simulink subsystem "SMC_Subsystem"  (R2023a)
settings: Solver=VariableStepAuto  StartTime=0.0  StopTime=10.0  RelTol=1e-3

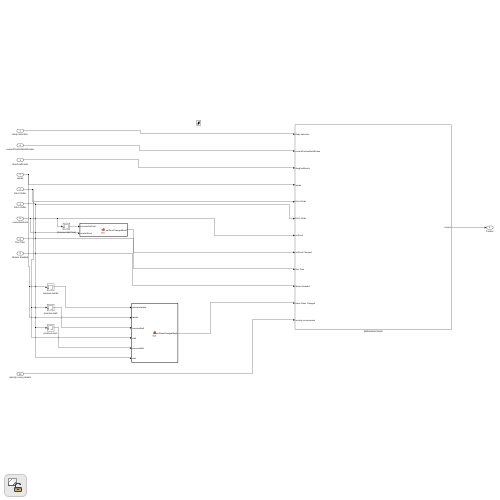
[thumbnail: Simulink's stored preview of the top-level diagram]
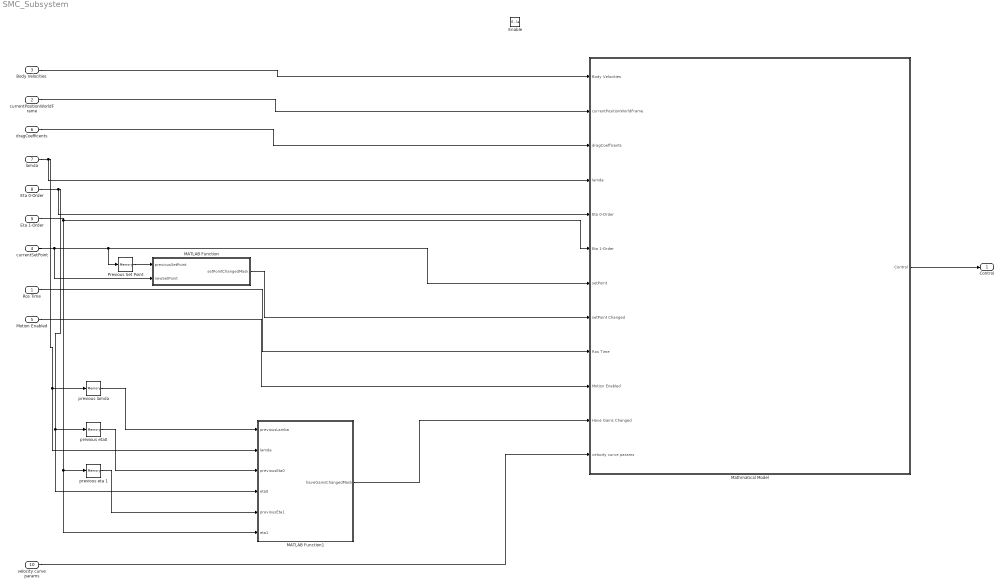
== system SMC_Subsystem ==
  Ros Time : Inport
  currentPositionWorldFrame : Inport  Port=2
  Body Velocities : Inport  Port=3
  currentSetPoint : Inport  Port=4
  Motion Enabled : Inport  Port=5
  dragCoefficents : Inport  Port=6
  lamda : Inport  Port=7
  Eta 0-Order : Inport  Port=8
  Eta 1-Order : Inport  Port=9
  velocity curve params : Inport  Port=10
  Enable : EnablePort
  MATLAB Function : MATLAB Function  TreatAsAtomicUnit=on
  MATLAB Function1 : MATLAB Function  TreatAsAtomicUnit=on
  Mathmatical Model : Subsystem
  Previous Set Point : Memory  InitialCondition=[0,0,0,0,0,0,0]  InheritSampleTime=on
  previous eta 1 : Memory  InheritSampleTime=on
  previous eta0 : Memory  InheritSampleTime=on
  previous lamda : Memory  InheritSampleTime=on
  Control : Outport
  wires:
  dragCoefficents/1 -> Mathmatical Model/3(dragCoefficents)
  Mathmatical Model/1(Control) -> Control/1
  currentSetPoint/1 -> Mathmatical Model/7(setPoint), Previous Set Point/1, MATLAB Function/2(newSetPoint)
  currentPositionWorldFrame/1 -> Mathmatical Model/2(currentPositionWorldFrame)
  Body Velocities/1 -> Mathmatical Model/1(Body Velocities)
  MATLAB Function/1(setPointChangedMask) -> Mathmatical Model/8(setPoint Changed)
  Previous Set Point/1 -> MATLAB Function/1(previousSetPoint)
  Ros Time/1 -> Mathmatical Model/9(Ros Time)
  Motion Enabled/1 -> Mathmatical Model/10(Motion Enabled)
  previous lamda/1 -> MATLAB Function1/1(previousLamba)
  previous eta0/1 -> MATLAB Function1/3(previousEta0)
  previous eta 1/1 -> MATLAB Function1/5(previousEta1)
  lamda/1 -> previous lamda/1, MATLAB Function1/2(lamda), Mathmatical Model/4(lamda)
  Eta 0-Order/1 -> MATLAB Function1/4(eta0), previous eta0/1, Mathmatical Model/5(Eta 0-Order)
  Eta 1-Order/1 -> Mathmatical Model/6(Eta 1-Order), MATLAB Function1/6(eta1), previous eta 1/1
  MATLAB Function1/1(haveGainsChangedMask) -> Mathmatical Model/11(Have Gains Changed)
  velocity curve params/1 -> Mathmatical Model/12(velocity curve params)

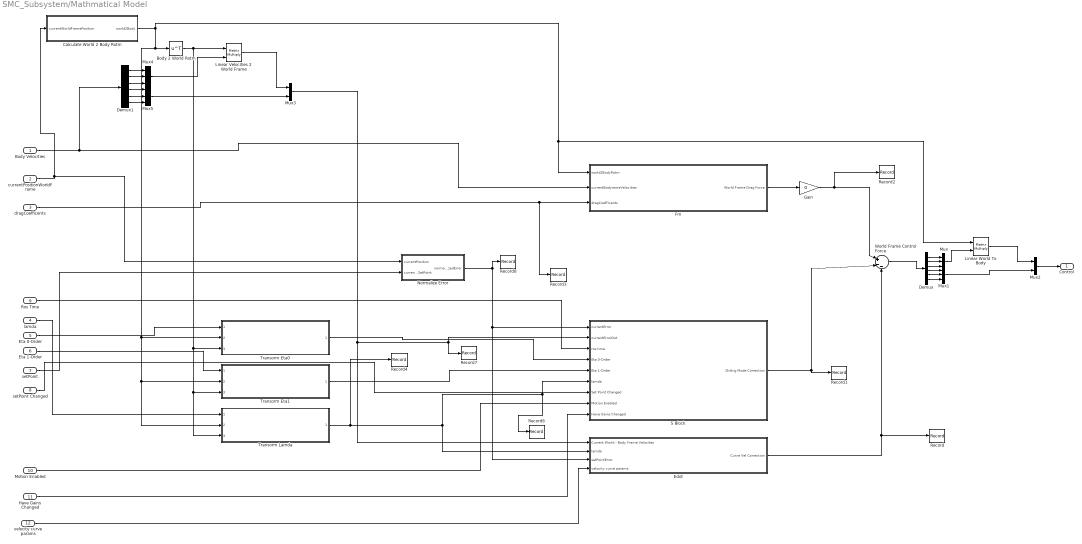
== system SMC_Subsystem/Mathmatical Model ==
  Body Velocities : Inport
  currentPositionWorldFrame : Inport  Port=2
  dragCoefficents : Inport  Port=3
  lamda : Inport  Port=4
  Eta 0-Order : Inport  Port=5
  Eta 1-Order : Inport  Port=6
  setPoint : Inport  Port=7
  setPoint Changed : Inport  Port=8
  Ros Time : Inport  Port=9
  Motion Enabled : Inport  Port=10
  Have Gains Changed : Inport  Port=11
  velocity curve params : Inport  Port=12
  Body 2 World Rotm : Math  Operator=transpose
  Calculate World 2 Body Rotm : MATLAB Function  TreatAsAtomicUnit=on
  Demux : Demux  Outputs=6
  Demux1 : Demux  Outputs=6
  Edot : Subsystem
  Fm : Subsystem
  Gain : Gain  Gain=0
  Linear Velocities 2 World Frame : Product  Multiplication=Matrix(*)
  Linear World To Body : Product  Multiplication=Matrix(*)
  Mux{,1,4..5} (4 alike) : Mux  Inputs=3
  Mux2 : Mux  Inputs=2
  Mux3 : Mux  Inputs=2
  Normalize Error : MATLAB Function  TreatAsAtomicUnit=on
  Record : Record  FileSettingsInternal="{\"entries\":[{\"content\":{\"excelSettings\":{\"content\":{},\"type\":\"Streamout.ExcelSettings\"}},\"type\":\"Streamout.FileSettingStorage\",\"uuid\":\"\"}],\"packageUris\":[\"http:\\/\\/schema.mathworks.com\\/mf0\\/streamout_blocks\\/R2020a\"],\"version\":\"1.0\"}"  Layout=[1 1]  SignalsInternal="{\"entries\":[{\"content\":{\"signals\":[{\"content\":{\"blockPath\":[],\"dimensions\":[6,1],\"domain\":\"\",\"hasChildren\":true,\"lineColor\":\"#b746ff\",\"port\":1,\"signalID\":2555,\"signalName\":\"Edot\"},\"type\":\"RecordBlkView.Signal\",\"uuid\":\"\"},{\"content\":{\"blockPath\":[],\"channel\":[1,1],\"dimensions\":[6,1],\"domain\":\"\",\"lineColor\":\"#4dbeee\",\"parentID\":2555,\"port\":1,\"signalID\":2556,\"signalName\":\"Edot\"},\"type\":\"RecordBlkView ...(+1172 chars)"  VisualizationBindings="{\"sparklinesplugin\":{\"info\":[{\"bindingParametersList\":[],\"subplotID\":1}]}}"
  Record1 : Record  FileSettingsInternal="{\"entries\":[{\"content\":{\"excelSettings\":{\"content\":{},\"type\":\"Streamout.ExcelSettings\"}},\"type\":\"Streamout.FileSettingStorage\",\"uuid\":\"\"}],\"packageUris\":[\"http:\\/\\/schema.mathworks.com\\/mf0\\/streamout_blocks\\/R2020a\"],\"version\":\"1.0\"}"  Layout=[1 1]  SignalsInternal="{\"entries\":[{\"content\":{\"signals\":[{\"content\":{\"blockPath\":[],\"dimensions\":[6,1],\"domain\":\"\",\"hasChildren\":true,\"lineColor\":\"#ff13a6\",\"port\":1,\"signalID\":2572,\"signalName\":\"S Block\"},\"type\":\"RecordBlkView.Signal\",\"uuid\":\"\"},{\"content\":{\"blockPath\":[],\"channel\":[1,1],\"dimensions\":[6,1],\"domain\":\"\",\"lineColor\":\"#0072bd\",\"parentID\":2572,\"port\":1,\"signalID\":2573,\"signalName\":\"S Block\"},\"type\":\"RecordB ...(+1193 chars)"  VisualizationBindings="{\"sparklinesplugin\":{\"info\":[{\"bindingParametersList\":[],\"subplotID\":1}]}}"
  Record2 : Record  FileSettingsInternal="{\"entries\":[{\"content\":{\"excelSettings\":{\"content\":{},\"type\":\"Streamout.ExcelSettings\"}},\"type\":\"Streamout.FileSettingStorage\",\"uuid\":\"\"}],\"packageUris\":[\"http:\\/\\/schema.mathworks.com\\/mf0\\/streamout_blocks\\/R2020a\"],\"version\":\"1.0\"}"  Layout=[1 1]  SignalsInternal="{\"entries\":[{\"content\":{\"signals\":[{\"content\":{\"blockPath\":[],\"dimensions\":[6],\"domain\":\"\",\"hasChildren\":true,\"lineColor\":\"#22b573\",\"port\":1,\"signalID\":2589,\"signalName\":\"Gain\"},\"type\":\"RecordBlkView.Signal\",\"uuid\":\"\"},{\"content\":{\"blockPath\":[],\"channel\":[1],\"dimensions\":[6],\"domain\":\"\",\"lineColor\":\"#edb120\",\"parentID\":2589,\"plots\":[1],\"port\":1,\"signalID\":2590,\"signalName\":\"Gain\"},\"type\":\"RecordB ...(+1206 chars)"  VisualizationBindings="{\"sparklinesplugin\":{\"info\":[{\"bindingParametersList\":[],\"subplotID\":1}]}}"
  Record3 : Record  FileSettingsInternal="{\"entries\":[{\"content\":{\"excelSettings\":{\"content\":{},\"type\":\"Streamout.ExcelSettings\"}},\"type\":\"Streamout.FileSettingStorage\",\"uuid\":\"\"}],\"packageUris\":[\"http:\\/\\/schema.mathworks.com\\/mf0\\/streamout_blocks\\/R2020a\"],\"version\":\"1.0\"}"  Layout=[1 1]  SignalsInternal="{\"entries\":[{\"content\":{\"signals\":[{\"content\":{\"blockPath\":[],\"dimensions\":[1,24],\"domain\":\"\",\"hasChildren\":true,\"lineColor\":\"#d95319\",\"port\":1,\"signalID\":2606,\"signalName\":\"dragCoefficents\"},\"type\":\"RecordBlkView.Signal\",\"uuid\":\"\"},{\"content\":{\"blockPath\":[],\"channel\":[1,1],\"dimensions\":[1,24],\"domain\":\"\",\"lineColor\":\"#77ac30\",\"parentID\":2606,\"plots\":[1],\"port\":1,\"signalID\":2607,\"signalName\":\"dra ...(+5141 chars)"  VisualizationBindings="{\"sparklinesplugin\":{\"info\":[{\"bindingParametersList\":[],\"subplotID\":1}]}}"
  Record4 : Record  FileSettingsInternal="{\"entries\":[{\"content\":{\"excelSettings\":{\"content\":{},\"type\":\"Streamout.ExcelSettings\"}},\"type\":\"Streamout.FileSettingStorage\",\"uuid\":\"\"}],\"packageUris\":[\"http:\\/\\/schema.mathworks.com\\/mf0\\/streamout_blocks\\/R2020a\"],\"version\":\"1.0\"}"  Layout=[1 1]  SignalsInternal="{\"entries\":[{\"content\":{\"signals\":[{\"content\":{\"blockPath\":[],\"dimensions\":[6],\"domain\":\"\",\"hasChildren\":true,\"lineColor\":\"#7e2f8e\",\"port\":1,\"signalID\":2659,\"signalName\":\"Transorm Lamda\"},\"type\":\"RecordBlkView.Signal\",\"uuid\":\"\"},{\"content\":{\"blockPath\":[],\"channel\":[1],\"dimensions\":[6],\"domain\":\"\",\"lineColor\":\"#64d413\",\"parentID\":2659,\"plots\":[1],\"port\":1,\"signalID\":2660,\"signalName\":\"Transorm Lam ...(+1276 chars)"  VisualizationBindings="{\"sparklinesplugin\":{\"info\":[{\"bindingParametersList\":[],\"subplotID\":1}]}}"
  Record6 : Record  FileSettingsInternal="{\"entries\":[{\"content\":{\"excelSettings\":{\"content\":{},\"type\":\"Streamout.ExcelSettings\"}},\"type\":\"Streamout.FileSettingStorage\",\"uuid\":\"\"}],\"packageUris\":[\"http:\\/\\/schema.mathworks.com\\/mf0\\/streamout_blocks\\/R2020a\"],\"version\":\"1.0\"}"  Layout=[1 1]  SignalsInternal="{\"entries\":[{\"content\":{\"signals\":[{\"content\":{\"blockPath\":[],\"dimensions\":[6],\"domain\":\"\",\"hasChildren\":true,\"lineColor\":\"#4dbeee\",\"port\":1,\"signalID\":2676,\"signalName\":\"Transorm Lamda\"},\"type\":\"RecordBlkView.Signal\",\"uuid\":\"\"},{\"content\":{\"blockPath\":[],\"channel\":[1],\"dimensions\":[6],\"domain\":\"\",\"lineColor\":\"#64d413\",\"parentID\":2676,\"plots\":[1],\"port\":1,\"signalID\":2677,\"signalName\":\"Transorm Lam ...(+1240 chars)"  VisualizationBindings="{\"sparklinesplugin\":{\"info\":[{\"bindingParametersList\":[],\"subplotID\":1}]}}"
  Record7 : Record  FileSettingsInternal="{\"entries\":[{\"content\":{\"excelSettings\":{\"content\":{},\"type\":\"Streamout.ExcelSettings\"}},\"type\":\"Streamout.FileSettingStorage\",\"uuid\":\"\"}],\"packageUris\":[\"http:\\/\\/schema.mathworks.com\\/mf0\\/streamout_blocks\\/R2020a\"],\"version\":\"1.0\"}"  Layout=[1 1]  SignalsInternal="{\"entries\":[{\"content\":{\"signals\":[{\"content\":{\"blockPath\":[],\"dimensions\":[6],\"domain\":\"\",\"hasChildren\":true,\"lineColor\":\"#139fff\",\"port\":1,\"signalID\":2693,\"signalName\":\"Mux3\"},\"type\":\"RecordBlkView.Signal\",\"uuid\":\"\"},{\"content\":{\"blockPath\":[],\"channel\":[1],\"dimensions\":[6],\"domain\":\"\",\"lineColor\":\"#edb120\",\"parentID\":2693,\"plots\":[1],\"port\":1,\"signalID\":2694,\"signalName\":\"Mux3\"},\"type\":\"RecordB ...(+1170 chars)"  VisualizationBindings="{\"sparklinesplugin\":{\"info\":[{\"bindingParametersList\":[],\"subplotID\":1}]}}"
  Record8 : Record  FileSettingsInternal="{\"entries\":[{\"content\":{\"excelSettings\":{\"content\":{},\"type\":\"Streamout.ExcelSettings\"}},\"type\":\"Streamout.FileSettingStorage\",\"uuid\":\"\"}],\"packageUris\":[\"http:\\/\\/schema.mathworks.com\\/mf0\\/streamout_blocks\\/R2020a\"],\"version\":\"1.0\"}"  Layout=[1 1]  SignalsInternal="{\"entries\":[{\"content\":{\"signals\":[{\"content\":{\"blockPath\":[],\"dimensions\":[1,6],\"domain\":\"\",\"hasChildren\":true,\"lineColor\":\"#b746ff\",\"port\":1,\"signalID\":2710,\"signalName\":\"Normalize Error\"},\"type\":\"RecordBlkView.Signal\",\"uuid\":\"\"},{\"content\":{\"blockPath\":[],\"channel\":[1,1],\"dimensions\":[1,6],\"domain\":\"\",\"lineColor\":\"#a2142f\",\"parentID\":2710,\"plots\":[1],\"port\":1,\"signalID\":2711,\"signalName\":\"Norma ...(+1273 chars)"  VisualizationBindings="{\"sparklinesplugin\":{\"info\":[{\"bindingParametersList\":[],\"subplotID\":1}]}}"
  S Block : Subsystem
  Transorm Eta0 : Subsystem  ReferencedSubsystem=Tranfsform_Linear_Gains_To_World
  Transorm Eta1 : Subsystem  ReferencedSubsystem=Tranfsform_Linear_Gains_To_World
  Transorm Lamda : Subsystem  ReferencedSubsystem=Tranfsform_Linear_Gains_To_World
  World Frame Control Force : Sum  Inputs=|+--
  Control : Outport
  wires:
  velocity curve params/1 -> Edot/4(velocity curve params)
  Have Gains Changed/1 -> S Block/9(Have Gains Changed)
  Motion Enabled/1 -> S Block/8(Motion Enabled)
  Transorm Eta0/1 -> S Block/4(Eta 0-Order)
  Body 2 World Rotm/1 -> Linear Velocities 2 World Frame/1, Transorm Lamda/3, Transorm Eta1/3, Transorm Eta0/3
  Edot/1(Curve Vel Correction) -> World Frame Control Force/3, Record/1
  Gain/1 -> World Frame Control Force/1, Record2/1
  Eta 1-Order/1 -> Transorm Eta1/1
  setPoint/1 -> Normalize Error/2(currentSetPoint)
  Normalize Error/1(normalizedError) -> S Block/1(currentError), Edot/3(setPointError), Record8/1
  Ros Time/1 -> S Block/3(ros time)
  setPoint Changed/1 -> S Block/7(Set Point Changed)
  Mux3/1 -> Edot/1(Current World - Body Frame Velocites), S Block/2(currentErrorDot), Record7/1
  Eta 0-Order/1 -> Transorm Eta0/1
  lamda/1 -> Transorm Lamda/1
  Transorm Eta1/1 -> S Block/5(Eta 1-Order)
  Transorm Lamda/1 -> Edot/2(lamda), S Block/6(lamda), Record6/1, Record4/1
  Mux5/1 -> Mux3/2
  Fm/1(World Frame Drag Force) -> Gain/1
  Demux1/6 -> Mux5/3
  Demux1/4 -> Mux5/1
  Demux1/5 -> Mux5/2
  Demux1/3 -> Mux4/3
  Demux1/1 -> Mux4/1
  Demux1/2 -> Mux4/2
  Mux4/1 -> Linear Velocities 2 World Frame/2
  Linear Velocities 2 World Frame/1 -> Mux3/1
  dragCoefficents/1 -> Fm/3(dragCoefficents), Record3/1
  Calculate World 2 Body Rotm/1(world2Body) -> Fm/1(world2BodyRotm), Linear World To Body/1, Transorm Lamda/2, Transorm Eta1/2, Transorm Eta0/2, Body 2 World Rotm/1
  Mux2/1 -> Control/1
  Mux1/1 -> Mux2/2
  Linear World To Body/1 -> Mux2/1
  Mux/1 -> Linear World To Body/2
  Demux/4 -> Mux1/1
  Demux/5 -> Mux1/2
  Demux/6 -> Mux1/3
  Demux/3 -> Mux/3
  Demux/2 -> Mux/2
  Demux/1 -> Mux/1
  World Frame Control Force/1 -> Demux/1
  S Block/1("Sliding Mode Correction ") -> Record1/1, World Frame Control Force/2
  currentPositionWorldFrame/1 -> Calculate World 2 Body Rotm/1(currentWorldFramePosition), Normalize Error/1(currentPosition)
  Body Velocities/1 -> Demux1/1, Fm/2(currentBodyrameVelocities)

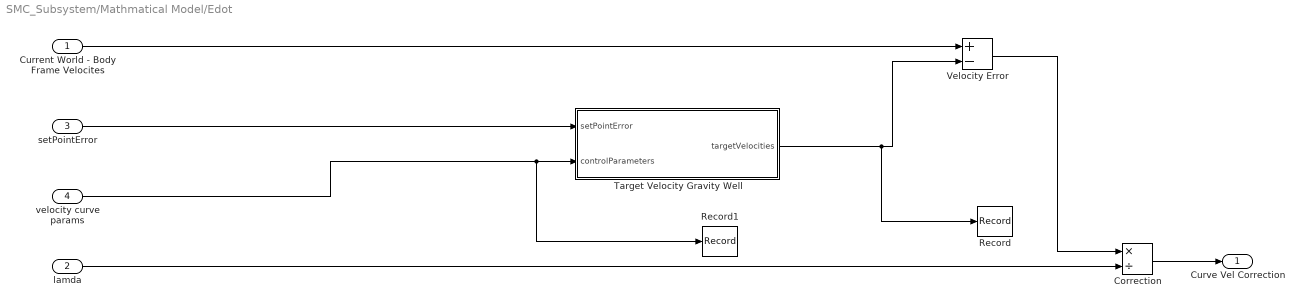
== system SMC_Subsystem/Mathmatical Model/Edot ==
  Current World - Body Frame Velocites : Inport
  lamda : Inport  Port=2
  setPointError : Inport  Port=3
  velocity curve params : Inport  Port=4
  Correction : Product  Inputs=*/
  Record : Record  FileSettingsInternal="{\"entries\":[{\"content\":{\"excelSettings\":{\"content\":{},\"type\":\"Streamout.ExcelSettings\"}},\"type\":\"Streamout.FileSettingStorage\",\"uuid\":\"\"}],\"packageUris\":[\"http:\\/\\/schema.mathworks.com\\/mf0\\/streamout_blocks\\/R2020a\"],\"version\":\"1.0\"}"  Layout=[1 1]  SignalsInternal="{\"entries\":[{\"content\":{\"signals\":[{\"content\":{\"blockPath\":[],\"dimensions\":[6,1],\"domain\":\"\",\"hasChildren\":true,\"lineColor\":\"#ff13a6\",\"port\":1,\"signalID\":2441,\"signalName\":\"Target Velocity Gravity Well\"},\"type\":\"RecordBlkView.Signal\",\"uuid\":\"\"},{\"content\":{\"blockPath\":[],\"channel\":[1,1],\"dimensions\":[6,1],\"domain\":\"\",\"lineColor\":\"#d95319\",\"parentID\":2441,\"plots\":[1],\"port\":1,\"signalID\":2442,\"signa ...(+1340 chars)"  VisualizationBindings="{\"sparklinesplugin\":{\"info\":[{\"bindingParametersList\":[],\"subplotID\":1}]}}"
  Record1 : Record  FileSettingsInternal="{\"entries\":[{\"content\":{\"excelSettings\":{\"content\":{},\"type\":\"Streamout.ExcelSettings\"}},\"type\":\"Streamout.FileSettingStorage\",\"uuid\":\"\"}],\"packageUris\":[\"http:\\/\\/schema.mathworks.com\\/mf0\\/streamout_blocks\\/R2020a\"],\"version\":\"1.0\"}"  Layout=[1 1]  SignalsInternal="{\"entries\":[{\"content\":{\"signals\":[{\"content\":{\"blockPath\":[],\"dimensions\":[1,12],\"domain\":\"\",\"hasChildren\":true,\"lineColor\":\"#22b573\",\"port\":1,\"signalID\":2458,\"signalName\":\"velocity curve params\"},\"type\":\"RecordBlkView.Signal\",\"uuid\":\"\"},{\"content\":{\"blockPath\":[],\"channel\":[1,1],\"dimensions\":[1,12],\"domain\":\"\",\"lineColor\":\"#edb120\",\"parentID\":2458,\"plots\":[1],\"port\":1,\"signalID\":2459,\"signalName ...(+2639 chars)"  VisualizationBindings="{\"sparklinesplugin\":{\"info\":[{\"bindingParametersList\":[],\"subplotID\":1}]}}"
  Target Velocity Gravity Well : MATLAB Function  TreatAsAtomicUnit=on
  Velocity Error : Sum  Inputs=+-
  Curve Vel Correction : Outport
  wires:
  velocity curve params/1 -> Target Velocity Gravity Well/2(controlParameters), Record1/1
  Target Velocity Gravity Well/1(targetVelocities) -> Velocity Error/2, Record/1
  setPointError/1 -> Target Velocity Gravity Well/1(setPointError)
  Velocity Error/1 -> Correction/1
  Current World - Body Frame Velocites/1 -> Velocity Error/1
  lamda/1 -> Correction/2
  Correction/1 -> Curve Vel Correction/1

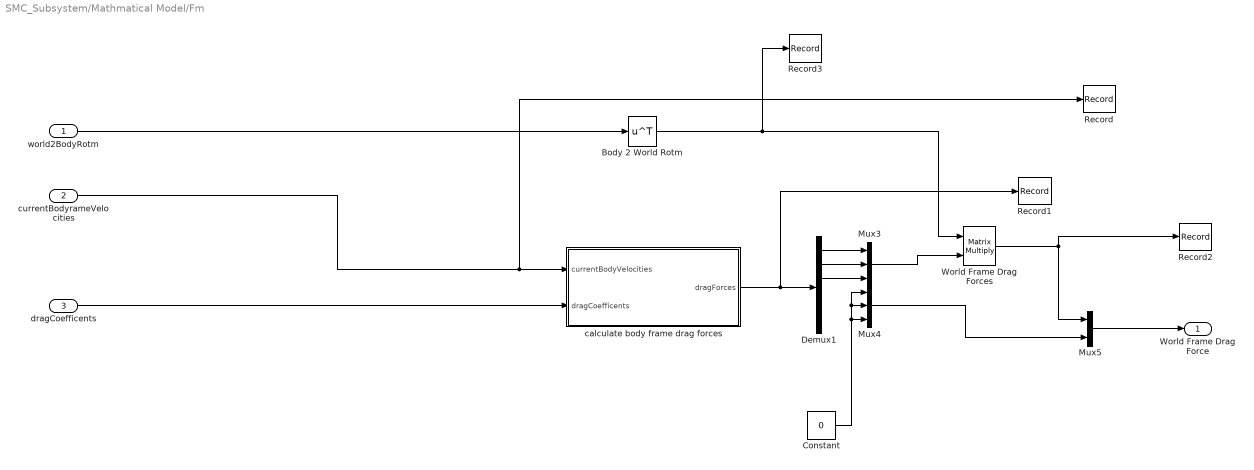
== system SMC_Subsystem/Mathmatical Model/Fm ==
  world2BodyRotm : Inport
  currentBodyrameVelocities : Inport  Port=2
  dragCoefficents : Inport  Port=3
  Body 2 World Rotm : Math  Operator=transpose
  Constant : Constant  Value=0
  Demux1 : Demux  Outputs=6
  Mux3 : Mux  Inputs=3
  Mux4 : Mux  Inputs=3
  Mux5 : Mux  Inputs=2
  Record : Record  FileSettingsInternal="{\"entries\":[{\"content\":{\"excelSettings\":{\"content\":{},\"type\":\"Streamout.ExcelSettings\"}},\"type\":\"Streamout.FileSettingStorage\",\"uuid\":\"\"}],\"packageUris\":[\"http:\\/\\/schema.mathworks.com\\/mf0\\/streamout_blocks\\/R2020a\"],\"version\":\"1.0\"}"  Layout=[1 1]  SignalsInternal="{\"entries\":[{\"content\":{\"signals\":[{\"content\":{\"blockPath\":[],\"dimensions\":[6],\"domain\":\"\",\"hasChildren\":true,\"lineColor\":\"#d95319\",\"port\":1,\"signalID\":2487,\"signalName\":\"currentBodyrameVelocities\"},\"type\":\"RecordBlkView.Signal\",\"uuid\":\"\"},{\"content\":{\"blockPath\":[],\"channel\":[1],\"dimensions\":[6],\"domain\":\"\",\"lineColor\":\"#b746ff\",\"parentID\":2487,\"plots\":[1],\"port\":1,\"signalID\":2488,\"signalName\":\"c ...(+1341 chars)"  VisualizationBindings="{\"sparklinesplugin\":{\"info\":[{\"bindingParametersList\":[],\"subplotID\":1}]}}"
  Record1 : Record  FileSettingsInternal="{\"entries\":[{\"content\":{\"excelSettings\":{\"content\":{},\"type\":\"Streamout.ExcelSettings\"}},\"type\":\"Streamout.FileSettingStorage\",\"uuid\":\"\"}],\"packageUris\":[\"http:\\/\\/schema.mathworks.com\\/mf0\\/streamout_blocks\\/R2020a\"],\"version\":\"1.0\"}"  Layout=[1 1]  SignalsInternal="{\"entries\":[{\"content\":{\"signals\":[{\"content\":{\"blockPath\":[],\"dimensions\":[6,1],\"domain\":\"\",\"hasChildren\":true,\"lineColor\":\"#7e2f8e\",\"port\":1,\"signalID\":2504,\"signalName\":\"calculate body frame drag forces\"},\"type\":\"RecordBlkView.Signal\",\"uuid\":\"\"},{\"content\":{\"blockPath\":[],\"channel\":[1,1],\"dimensions\":[6,1],\"domain\":\"\",\"lineColor\":\"#139fff\",\"parentID\":2504,\"plots\":[1],\"port\":1,\"signalID\":2505,\"s ...(+1428 chars)"  VisualizationBindings="{\"sparklinesplugin\":{\"info\":[{\"bindingParametersList\":[],\"subplotID\":1}]}}"
  Record2 : Record  FileSettingsInternal="{\"entries\":[{\"content\":{\"excelSettings\":{\"content\":{},\"type\":\"Streamout.ExcelSettings\"}},\"type\":\"Streamout.FileSettingStorage\",\"uuid\":\"\"}],\"packageUris\":[\"http:\\/\\/schema.mathworks.com\\/mf0\\/streamout_blocks\\/R2020a\"],\"version\":\"1.0\"}"  SignalsInternal="{\"entries\":[{\"content\":{\"signals\":[{\"content\":{\"blockPath\":[],\"dimensions\":[3],\"domain\":\"\",\"hasChildren\":true,\"lineColor\":\"#4dbeee\",\"port\":1,\"signalID\":2521,\"signalName\":\"World Frame Drag Forces\"},\"type\":\"RecordBlkView.Signal\",\"uuid\":\"\"},{\"content\":{\"blockPath\":[],\"channel\":[1],\"dimensions\":[3],\"domain\":\"\",\"lineColor\":\"#b746ff\",\"parentID\":2521,\"plots\":[1],\"port\":1,\"signalID\":2522,\"signalName\":\"Wor ...(+661 chars)"  VisualizationBindings="{\"sparklinesplugin\":{\"info\":[{\"bindingParametersList\":[],\"subplotID\":1}]}}"
  Record3 : Record  FileSettingsInternal="{\"entries\":[{\"content\":{\"excelSettings\":{\"content\":{},\"type\":\"Streamout.ExcelSettings\"}},\"type\":\"Streamout.FileSettingStorage\",\"uuid\":\"\"}],\"packageUris\":[\"http:\\/\\/schema.mathworks.com\\/mf0\\/streamout_blocks\\/R2020a\"],\"version\":\"1.0\"}"  Layout=[1 1]  SignalsInternal="{\"entries\":[{\"content\":{\"signals\":[{\"content\":{\"blockPath\":[],\"dimensions\":[3,3],\"domain\":\"\",\"hasChildren\":true,\"lineColor\":\"#139fff\",\"port\":1,\"signalID\":2532,\"signalName\":\"Body 2 World Rotm\"},\"type\":\"RecordBlkView.Signal\",\"uuid\":\"\"},{\"content\":{\"blockPath\":[],\"channel\":[1,1],\"dimensions\":[3,3],\"domain\":\"\",\"lineColor\":\"#a2142f\",\"parentID\":2532,\"plots\":[1],\"port\":1,\"signalID\":2533,\"signalName\":\"Bod ...(+1995 chars)"  VisualizationBindings="{\"sparklinesplugin\":{\"info\":[{\"bindingParametersList\":[],\"subplotID\":1}]}}"
  World Frame Drag Forces : Product  Multiplication=Matrix(*)
  calculate body frame drag forces : MATLAB Function  TreatAsAtomicUnit=on
  World Frame Drag Force : Outport
  wires:
  Constant/1 -> Mux4/1, Mux4/2, Mux4/3
  Mux4/1 -> Mux5/2
  calculate body frame drag forces/1(dragForces) -> Demux1/1, Record1/1
  Body 2 World Rotm/1 -> World Frame Drag Forces/1, Record3/1
  world2BodyRotm/1 -> Body 2 World Rotm/1
  dragCoefficents/1 -> calculate body frame drag forces/2(dragCoefficents)
  currentBodyrameVelocities/1 -> calculate body frame drag forces/1(currentBodyVelocities), Record/1
  Demux1/2 -> Mux3/2
  Mux5/1 -> World Frame Drag Force/1
  Demux1/3 -> Mux3/3
  Mux3/1 -> World Frame Drag Forces/2
  Demux1/1 -> Mux3/1
  World Frame Drag Forces/1 -> Record2/1, Mux5/1

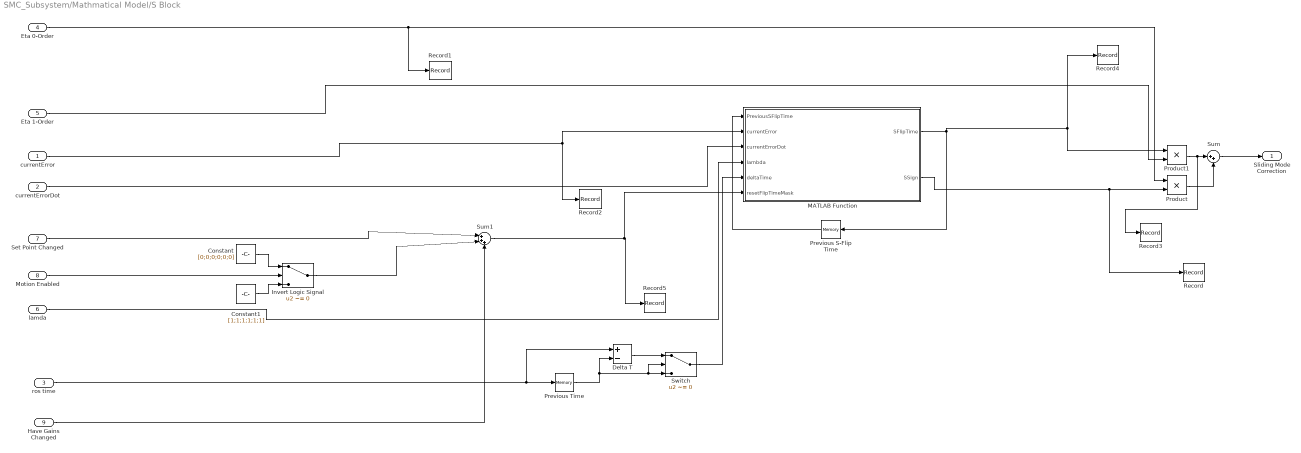
== system SMC_Subsystem/Mathmatical Model/S Block ==
  currentError : Inport
  currentErrorDot : Inport  Port=2
  ros time : Inport  Port=3
  Eta 0-Order : Inport  Port=4
  Eta 1-Order : Inport  Port=5
  lamda : Inport  Port=6
  Set Point Changed : Inport  Port=7
  Motion Enabled : Inport  Port=8
  Have Gains Changed : Inport  Port=9
  Constant : Constant  Value=[0;0;0;0;0;0]
  Constant1 : Constant  Value=[1;1;1;1;1;1]
  Delta T : Sum  Inputs=+-
  Invert Logic Signal : Switch  Criteria=u2 ~= 0  SaturateOnIntegerOverflow=off  InputSameDT=off
  MATLAB Function : MATLAB Function  TreatAsAtomicUnit=on
  Previous S-Flip Time : Memory  InitialCondition=[0;0;0;0;0;0]  InheritSampleTime=on
  Previous Time : Memory  InheritSampleTime=on
  Product : Product
  Product1 : Product
  Record : Record  FileSettingsInternal="{\"entries\":[{\"content\":{\"excelSettings\":{\"content\":{},\"type\":\"Streamout.ExcelSettings\"}},\"type\":\"Streamout.FileSettingStorage\",\"uuid\":\"\"}],\"packageUris\":[\"http:\\/\\/schema.mathworks.com\\/mf0\\/streamout_blocks\\/R2020a\"],\"version\":\"1.0\"}"  Layout=[1 1]  SignalsInternal="{\"entries\":[{\"content\":{\"signals\":[{\"content\":{\"blockPath\":[],\"dimensions\":[6,1],\"domain\":\"\",\"hasChildren\":true,\"lineColor\":\"#b746ff\",\"port\":1,\"signalID\":2727,\"signalName\":\"MATLAB Function:2\"},\"type\":\"RecordBlkView.Signal\",\"uuid\":\"\"},{\"content\":{\"blockPath\":[],\"channel\":[1,1],\"dimensions\":[6,1],\"domain\":\"\",\"lineColor\":\"#77ac30\",\"parentID\":2727,\"plots\":[1],\"port\":1,\"signalID\":2728,\"signalName\":\"MAT ...(+1287 chars)"  VisualizationBindings="{\"sparklinesplugin\":{\"info\":[{\"bindingParametersList\":[],\"subplotID\":1}]}}"
  Record1 : Record  FileSettingsInternal="{\"entries\":[{\"content\":{\"excelSettings\":{\"content\":{},\"type\":\"Streamout.ExcelSettings\"}},\"type\":\"Streamout.FileSettingStorage\",\"uuid\":\"\"}],\"packageUris\":[\"http:\\/\\/schema.mathworks.com\\/mf0\\/streamout_blocks\\/R2020a\"],\"version\":\"1.0\"}"  Layout=[1 1]  SignalsInternal="{\"entries\":[{\"content\":{\"signals\":[{\"content\":{\"blockPath\":[],\"dimensions\":[6],\"domain\":\"\",\"hasChildren\":true,\"lineColor\":\"#ff13a6\",\"port\":1,\"signalID\":2744,\"signalName\":\"Eta 0-Order\"},\"type\":\"RecordBlkView.Signal\",\"uuid\":\"\"},{\"content\":{\"blockPath\":[],\"channel\":[1],\"dimensions\":[6],\"domain\":\"\",\"lineColor\":\"#a2142f\",\"parentID\":2744,\"plots\":[1],\"port\":1,\"signalID\":2745,\"signalName\":\"Eta 0-Order\"},\" ...(+1219 chars)"  VisualizationBindings="{\"sparklinesplugin\":{\"info\":[{\"bindingParametersList\":[],\"subplotID\":1}]}}"
  Record2 : Record  FileSettingsInternal="{\"entries\":[{\"content\":{\"excelSettings\":{\"content\":{},\"type\":\"Streamout.ExcelSettings\"}},\"type\":\"Streamout.FileSettingStorage\",\"uuid\":\"\"}],\"packageUris\":[\"http:\\/\\/schema.mathworks.com\\/mf0\\/streamout_blocks\\/R2020a\"],\"version\":\"1.0\"}"  Layout=[1 1]  SignalsInternal="{\"entries\":[{\"content\":{\"signals\":[{\"content\":{\"blockPath\":[],\"dimensions\":[1,6],\"domain\":\"\",\"hasChildren\":true,\"lineColor\":\"#22b573\",\"port\":1,\"signalID\":2761,\"signalName\":\"currentError\"},\"type\":\"RecordBlkView.Signal\",\"uuid\":\"\"},{\"content\":{\"blockPath\":[],\"channel\":[1,1],\"dimensions\":[1,6],\"domain\":\"\",\"lineColor\":\"#7e2f8e\",\"parentID\":2761,\"plots\":[1],\"port\":1,\"signalID\":2762,\"signalName\":\"currentE ...(+1252 chars)"  VisualizationBindings="{\"sparklinesplugin\":{\"info\":[{\"bindingParametersList\":[],\"subplotID\":1}]}}"
  Record3 : Record  FileSettingsInternal="{\"entries\":[{\"content\":{\"excelSettings\":{\"content\":{},\"type\":\"Streamout.ExcelSettings\"}},\"type\":\"Streamout.FileSettingStorage\",\"uuid\":\"\"}],\"packageUris\":[\"http:\\/\\/schema.mathworks.com\\/mf0\\/streamout_blocks\\/R2020a\"],\"version\":\"1.0\"}"  Layout=[1 1]  SignalsInternal="{\"entries\":[{\"content\":{\"signals\":[{\"content\":{\"blockPath\":[],\"dimensions\":[6,1],\"domain\":\"\",\"hasChildren\":true,\"lineColor\":\"#d95319\",\"port\":1,\"signalID\":2778,\"signalName\":\"Product1\"},\"type\":\"RecordBlkView.Signal\",\"uuid\":\"\"},{\"content\":{\"blockPath\":[],\"channel\":[1,1],\"dimensions\":[6,1],\"domain\":\"\",\"lineColor\":\"#b746ff\",\"parentID\":2778,\"plots\":[1],\"port\":1,\"signalID\":2779,\"signalName\":\"Product1\"},\" ...(+1224 chars)"  VisualizationBindings="{\"sparklinesplugin\":{\"info\":[{\"bindingParametersList\":[],\"subplotID\":1}]}}"
  Record4 : Record  FileSettingsInternal="{\"entries\":[{\"content\":{\"excelSettings\":{\"content\":{},\"type\":\"Streamout.ExcelSettings\"}},\"type\":\"Streamout.FileSettingStorage\",\"uuid\":\"\"}],\"packageUris\":[\"http:\\/\\/schema.mathworks.com\\/mf0\\/streamout_blocks\\/R2020a\"],\"version\":\"1.0\"}"  Layout=[1 1]  SignalsInternal="{\"entries\":[{\"content\":{\"signals\":[{\"content\":{\"blockPath\":[],\"dimensions\":[6,1],\"domain\":\"\",\"hasChildren\":true,\"lineColor\":\"#7e2f8e\",\"port\":1,\"signalID\":2795,\"signalName\":\"MATLAB Function:1\"},\"type\":\"RecordBlkView.Signal\",\"uuid\":\"\"},{\"content\":{\"blockPath\":[],\"channel\":[1,1],\"dimensions\":[6,1],\"domain\":\"\",\"lineColor\":\"#4dbeee\",\"parentID\":2795,\"plots\":[1],\"port\":1,\"signalID\":2796,\"signalName\":\"MAT ...(+1275 chars)"  VisualizationBindings="{\"sparklinesplugin\":{\"info\":[{\"bindingParametersList\":[],\"subplotID\":1}]}}"
  Record5 : Record  FileSettingsInternal="{\"entries\":[{\"content\":{\"excelSettings\":{\"content\":{},\"type\":\"Streamout.ExcelSettings\"}},\"type\":\"Streamout.FileSettingStorage\",\"uuid\":\"\"}],\"packageUris\":[\"http:\\/\\/schema.mathworks.com\\/mf0\\/streamout_blocks\\/R2020a\"],\"version\":\"1.0\"}"  Layout=[1 1]  SignalsInternal="{\"entries\":[{\"content\":{\"signals\":[{\"content\":{\"blockPath\":[],\"dimensions\":[1,6],\"domain\":\"\",\"hasChildren\":true,\"lineColor\":\"#4dbeee\",\"port\":1,\"signalID\":2812,\"signalName\":\"Sum1\"},\"type\":\"RecordBlkView.Signal\",\"uuid\":\"\"},{\"content\":{\"blockPath\":[],\"channel\":[1,1],\"dimensions\":[1,6],\"domain\":\"\",\"lineColor\":\"#ff13a6\",\"parentID\":2812,\"plots\":[1],\"port\":1,\"signalID\":2813,\"signalName\":\"Sum1\"},\"type\":\"R ...(+1184 chars)"  VisualizationBindings="{\"sparklinesplugin\":{\"info\":[{\"bindingParametersList\":[],\"subplotID\":1}]}}"
  Sum : Sum  Inputs=|++
  Sum1 : Sum  Inputs=|+++
  Switch : Switch  Criteria=u2 ~= 0  SaturateOnIntegerOverflow=off  InputSameDT=off
  "Sliding Mode Correction " : Outport
  wires:
  Invert Logic Signal/1 -> Sum1/2
  Have Gains Changed/1 -> Sum1/3
  Delta T/1 -> Switch/1
  Switch/1 -> MATLAB Function/5(deltaTime)
  ros time/1 -> Delta T/1, Previous Time/1
  Previous Time/1 -> Delta T/2, Switch/3, Switch/2
  Constant1/1 -> Invert Logic Signal/3
  Constant/1 -> Invert Logic Signal/1
  Motion Enabled/1 -> Invert Logic Signal/2
  Set Point Changed/1 -> Sum1/1
  Sum1/1 -> Record5/1, MATLAB Function/6(resetFlipTimeMask)
  lamda/1 -> MATLAB Function/4(lambda)
  Eta 1-Order/1 -> Product1/2
  Eta 0-Order/1 -> Product/1, Record1/1
  Previous S-Flip Time/1 -> MATLAB Function/1(PreviousSFlipTime)
  Sum/1 -> "Sliding Mode Correction "/1
  MATLAB Function/1(SFlipTime) -> Previous S-Flip Time/1, Product1/1, Record4/1
  Product1/1 -> Sum/1, Record3/1
  Product/1 -> Sum/2
  currentError/1 -> Record2/1, MATLAB Function/2(currentError)
  currentErrorDot/1 -> MATLAB Function/3(currentErrorDot)
  MATLAB Function/2(SSign) -> Product/2, Record/1

== matlab function SMC_Subsystem/MATLAB Function ==
function setPointChangedMask = fcn(previousSetPoint, newSetPoint)

setPointChangedMask = zeros(1,6);

%determine wether or not the set point has chnaged - element wise

previousEulerSetPoint = [previousSetPoint(1), previousSetPoint(2), previousSetPoint(3), quat2eul([previousSetPoint(7), previousSetPoint(4), previousSetPoint(5), previousSetPoint(6)])];
newEulerSetPoint = [newSetPoint(1), newSetPoint(2), newSetPoint(3), quat2eul([newSetPoint(7), newSetPoint(4), newSetPoint(5), newSetPoint(6)])];

%not changed = 0, true - everything else
setPointChangedMask = abs(previousEulerSetPoint - newEulerSetPoint);

%allow buffer on angular to account for slight shift due to conversion
%error...
for i=4:6
    if(setPointChangedMask(i) < .1)
        setPointChangedMask(i) = 0;
    end

    %catch nans and reset if they occur
    if(isnan(setPointChangedMask(i)))
        setPointChangedMask(i) = 1;
    end
end

== matlab function SMC_Subsystem/MATLAB Function1 ==
function haveGainsChangedMask = fcn(previousLamba, lamda, previousEta0, eta0, previousEta1, eta1)

%determine wether or not the set point has chnaged element wise
haveGainsChangedMask = abs(previousLamba - lamda) + abs(previousEta0 - eta0) + abs(previousEta1 - eta1);

== matlab function SMC_Subsystem/Mathmatical Model/Calculate World 2 Body Rotm ==
function world2Body = fcn(currentWorldFramePosition)

%convert ros2 quat to matlab quat - quat is last 
quat = [currentWorldFramePosition(7), currentWorldFramePosition(4), currentWorldFramePosition(5), currentWorldFramePosition(6)];

%calculate the rotation matrix representing the current orientation
world2Body = quat2rotm(quat);

%matlab issue
world2Body = transpose(world2Body);

== matlab function SMC_Subsystem/Mathmatical Model/Edot/Target Velocity Gravity Well ==
function targetVelocities = fcn(setPointError, controlParameters)

%the target velocities to converge to 
targetVelocities = zeros(6,1);

controlParametersExpectedLength = 12;
if(~length(controlParameters) == controlParametersExpectedLength)
    %params have not yet been assigned / assgined incorrectly
    return
end

controlParameters = reshape(controlParameters, [length(controlParameters) / 6, 6]);
%param(1,x) = max control value
%param(2,x) = the error where max control is reached

%velocity curves = param(1,x) * (-cos(error * pi / (2 * param(2,x)))^1/2 + 1)
for i=1:6
    if(controlParameters(2, i) == 0 || setPointError(i) == 0)
        targetVelocities(i) = 0;
    else
        %ensure the saturation error is not exceeded
        if(abs(setPointError(i)) > controlParameters(2, i))
            setPointError(i) = controlParameters(2, i) * setPointError(i) / abs(setPointError(i));
        end

        targetVelocities(i) = controlParameters(1,i) * (-cos(setPointError(i) * pi / (2 * controlParameters(2,i)))^(1/2) + 1);

        %enforce sign
        targetVelocities(i) = -(targetVelocities(i)) * setPointError(i) / abs(setPointError(i));
    end


end

== matlab function SMC_Subsystem/Mathmatical Model/Fm/calculate body frame drag forces ==
function dragForces = fcn(currentBodyVelocities, dragCoefficents)

dragForces = zeros(6,1);

expectedDragCoefficentLength = 24;
if(expectedDragCoefficentLength ~= length(dragCoefficents))
    %drag coefficents are not the expected length
    return 
end

%reshape drag coefficents array into a more sensible form
dc = reshape(dragCoefficents, [expectedDragCoefficentLength / 6, 6]);

for i=1:6
    %calculate the forces created by drag
    dragForces(i) = dc(1, i) + abs(currentBodyVelocities(i)) * dc(2, i) + exp(abs(currentBodyVelocities(i)) / dc(4, i))* dc(3, i);

    %take into account sign
    sign = 0;
    if(currentBodyVelocities(i) ~= 0)
        sign = currentBodyVelocities(i) / abs(currentBodyVelocities(i));
    end

    dragForces(i) = sign * dragForces(i);
end

== matlab function SMC_Subsystem/Mathmatical Model/Normalize Error ==
function normalizedError = fcn(currentPosition, currentSetPoint)

normalized = zeros(1,6);

normalized(1) = currentPosition(1) - currentSetPoint(1);
normalized(2) = currentPosition(2) - currentSetPoint(2);
normalized(3) = currentPosition(3) - currentSetPoint(3);

W2B = [currentPosition(7), currentPosition(4), currentPosition(5), currentPosition(6)];
setQuat = [currentSetPoint(7), -currentSetPoint(4), -currentSetPoint(5), -currentSetPoint(6)];


%Talos Heading in Body Frame
Tbody = [1,0,0,0];

%Transform from Body 2 World
B2W = [W2B(1), -W2B(2), -W2B(3), -W2B(4)] / (norm(W2B) ^ 2);

%Talos Heading in World Frame
TWorld = quatmultiply(Tbody, B2W);

%Talos Heading in World Frame Conjugate
TWorldI = [TWorld(1), -TWorld(2), -TWorld(3), -TWorld(4)];

%Current Yaw Error
eQuat = quatmultiply(setQuat, TWorldI);

% %axis Error
axisError = [eQuat(2), eQuat(3), eQuat(4)];
if(eQuat(1) < 0)
    axisError = -axisError;
end


normalized(4) = axisError(1);
normalized(5) = axisError(2);
normalized(6) = axisError(3);

normalizedError = normalized;

== matlab function SMC_Subsystem/Mathmatical Model/S Block/MATLAB Function ==
function [SFlipTime, SSign] = fcn(PreviousSFlipTime, currentError, currentErrorDot, lambda, deltaTime, resetFlipTimeMask)

%FlipTime, SSign and Previous are 6 by arrays - 1 per dof

SFlipTime = PreviousSFlipTime;
SSign = zeros(6,1);

%calculate S
S = currentError + lambda' .* currentErrorDot';


%just so nothing explodes - ill be impressed if this happens
for i=1:6

    %ensure no S equals zero
    if(S(i) == 0)
        SSign(i) = 0;
    else
        SSign(i) = S(i) / abs(S(i));
    end
end


%see if Sdot has flipped
for i=1:6

    %if the flip time is not to be reset
    if(~resetFlipTimeMask(i))
        if(SFlipTime(i) * SSign(i) > 0)
            SFlipTime(i) = SFlipTime(i) + deltaTime * SSign(i);
        else
            SFlipTime(i) = deltaTime * SSign(i);
        end
    else
       SFlipTime(i) = 0;
    end
end
